simulink model "SP_SImulink_Pavan"  (R2021b)
settings: Solver=VariableStepAuto  StartTime=0.0  StopTime=10  RelTol=1e-3
undefined symbols (not defined in the file or in its folder): g, k, l, theta, w
settings Model: Creator=Pavan Sandaka  LastModifiedBy=Pavan Sandaka

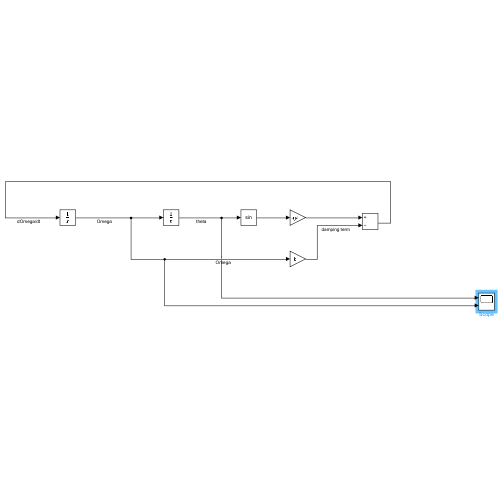
[thumbnail: Simulink's stored preview of the top-level diagram]
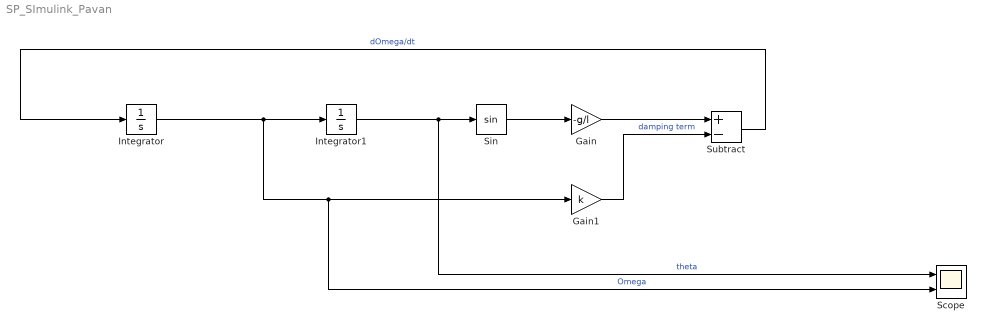
== system SP_SImulink_Pavan ==
  Gain : Gain  Gain=-g/l
  Gain1 : Gain  Gain=k
  Integrator : Integrator  InitialCondition=w
  Integrator1 : Integrator  InitialCondition=theta
  Scope : Scope  NumInputPorts=2
  Sin : Trigonometry
  Subtract : Sum  Inputs=+-
  wires:
  Subtract/1 -> Integrator/1  "dOmega/dt"
  Integrator/1 -> Scope/2, Gain1/1, Integrator1/1  "Omega"
  Integrator1/1 -> Scope/1, Sin/1  "theta"
  Sin/1 -> Gain/1
  Gain/1 -> Subtract/1
  Gain1/1 -> Subtract/2  "damping term"
